simulink library "FAS"  (R2022b)
settings: Solver=VariableStepAuto  StartTime=0.0  StopTime=10.0  RelTol=1e-3
undefined symbols (not defined in the file or in its folder): FASAppl, FASComp
libraries: FasBtc x2
settings Model: Creator=sk1042978  LastModifiedBy=kl13806
settings SolverCC: AlgebraicLoopSolver=TrustRegion
settings DebuggingCC: UnconnectedInputMsg=warning  UnconnectedOutputMsg=warning  UnconnectedLineMsg=warning  SFMachineParentedDataDiag=warning
settings ModelReferenceCC: EnableRefExpFcnMdlSchedulingChecks=on
settings RTWCC: DLArmComputeVersion=19.05

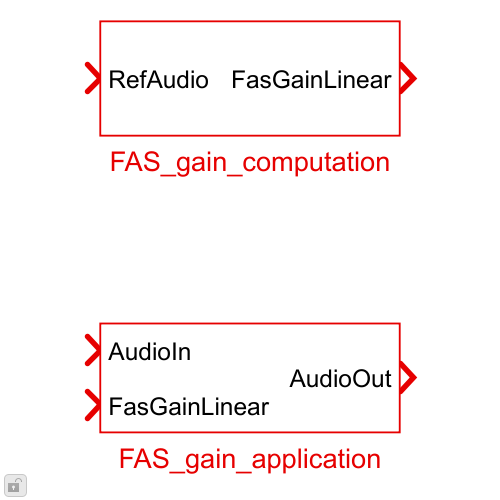
[thumbnail: Simulink's stored preview of the top-level diagram]
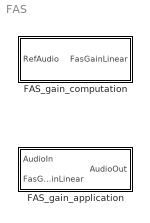
== system FAS ==
  FAS_gain_application : Subsystem  mask(Bose Fresh Air Speakers - Gain Application){MaskFasEnable=[ones(10,1)' zeros(6,1)'], MaskFASConfig=FASAppl, MaskDefaultFlag=on}
      mask prompts: MaskFasEnable "FAS enable"; MaskFASConfig "Configuration"; MaskDefaultFlag "Use default configuration"
      mask help:
      | The Fresh Air Speaker (FAS) algorithm is designed to limit the output level of selected speaker channels. The level of the remaining channels remains unaffected. This has been implemented in 2 parts - a FAS gain computation block and a FAS gain application block. Refer to the Help section for more information.
      |
      | This limiting is only necessary when windows are open, leading to a reduction in the excursion range of the FAS transducers in order to prevent damage.
      mask init:
      | blkh = gcbh;
      | 
      | % Clobber the configuration if the default values are desired
      | if (MaskDefaultFlag)
      |     MaskFASConfig = [];
      | end
      | MaskFASConfig = BTConfig.Assert('FASApplicationConfig',MaskFASConfig);
      | 
      | % Copy from MaskFASConfig to FasGainApplicationConfig
      | InnerLinkConfig = FasGainApplicationConfig;
      | InnerLinkConfig.DefaultLpfTimeConstMsec = MaskFASConfig.lpfTimeConstMsec;
      | 
      | % Copy the (previously) promoted TuneVar default to BTC
      | InnerLinkConfig.DefautFasEnable = MaskFasEnable;
      mask Help:
      | FAS Gain Application:
      | Description:
      | Applies the gain factor to the incoming audio after ramping it using a LPF. Inputs to the block are the gain factor (at framerate) and the input audio. Output from the block is the audio with the gain factors applied.
      | 
      | Mask parameters:
      | 1. FAS enable for each channel (uint32 ; [numChannels x 1]) - Either 0/1 (FAS disable/enable). Will throw an error if number of input audio channels does not match this array size.
      | 2. System parameters like frame size and sample rate are extracted from the input audio.
      | 3. Configuration: The default configuration is defined in FASApplicationConfig.m (FAS computation has a separate configuration file). Please check the file for more details on how to modify the default values.
      | 
      | Tuning support:
      | 1. LPF cut-off frequency - (Hz ; single) Ramps the gain factor
      | 2. FAS enable for each channel - (uint32) Promoted as a mask parameter
      mask Callback MaskDefaultFlag: FASMask.DefaultFlagCallback(gcbh,'MaskDefaultFlag','MaskFASConfig');
  FAS_gain_computation : Subsystem  mask(Bose Fresh Air Speakers - Gain Computation){MaskFASConfig=FASComp, MaskDefaultFlag=on}
      mask prompts: MaskFASConfig "Configuration"; MaskDefaultFlag "Use default configuration"
      mask help:
      | The Fresh Air Speaker (FAS) algorithm is designed to limit the output level of selected speaker channels. The output level of the remaining channels remains unaffected. This has been implemented in 2 parts - a FAS gain computation block and a FAS gain application block. The audio input to this block is only used to get audio stats (which will define the samplerate of this block).
      |
      | This limiting is only necessary when windows are open, leading to a reduction in the excursion range of the FAS transducers in order to prevent damage.
      mask init:
      | blkh = gcbh;
      | 
      | % Clobber the configuration if the default values are desired
      | if (MaskDefaultFlag)
      |     MaskFASConfig = [];
      | end
      | MaskFASConfig = BTConfig.Assert('FASComputationConfig',MaskFASConfig);
      | 
      | % Copy from MaskFASConfig to FasGainComputationConfig
      | InnerLinkConfig = FasGainComputationConfig;
      | InnerLinkConfig.DefaultSpeedGainSlope = MaskFASConfig.SpeedGainSlope;
      | InnerLinkConfig.DefaultSpeedGainThreshold = MaskFASConfig.SpeedGainThreshold;
      | InnerLinkConfig.DefaultGainMinValue = MaskFASConfig.GainMinValue;
      | InnerLinkConfig.DefaultSlewAttackDbPerSec = MaskFASConfig.slew_attackdBperSec;
      | InnerLinkConfig.DefaulySlewDecayDbPerSec = MaskFASConfig.slew_decaydBperSec;
      | InnerLinkConfig.DefaultSlewSlowDbPerSec = MaskFASConfig.slew_slowSlewdBperSec;
      | InnerLinkConfig.DefaultSlewThreshold = MaskFASConfig.slew_threshold;
      mask Help:
      | FAS Gain computation:
      | Description:
      | Computes the gain factor (based on speed and window status) to be applied to the channels which need pressure protection. Speed input is to be provided (either from the AudioPilot block or from a standalone RTC). The output gain factor is a value between [0,1]. System parameters like frame size and sample rate need to be provided through the mask.
      | 
      | Mask parameters:
      | 1. Configuration: The default configuration is defined in FASComputationConfig.m (FASApplication has a separate configuration file). Please check the file for more details on how to modify the default configuration.
      | 
      | Control support :
      | 1. Window Open status - (uint32) Can be 0 (window not open, FAS not needed) or 1 (window open, FAS needed).
      | 2. Speed In - (single) Current speed of the vehicle
      | 
      | Tuning support:
      | 1. Log minimum value - (single) To ensure that the computed gain in dB does not go to zero
      | 2. Slew Attack - (dB/second) Controls how fast the gain factor increases. TOP is specified in dB/samples.
      | 3. Slew Decay - (dB/second) Controls how fast the gain factor decreases. TOP is specified in dB/samples.
      | 4. Slew Threshold - (dB) If the change in slew is within this threshold, there is no update.
      | 5. Slow slew- (dB/second) Can be ignored for FAS.
      | 6. Speed Threshold (speed units) - Speed beyond which a negative gain is applied
      | 7. Speed Slope - Slope which the speed curve follows for the gain reduction.
      mask Callback MaskDefaultFlag: FASMask.DefaultFlagCallback(gcbh,'MaskDefaultFlag','MaskFASConfig');

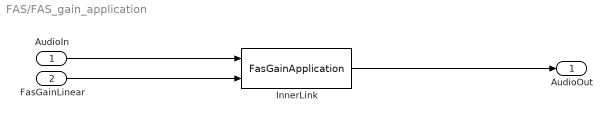
== system FAS/FAS_gain_application ==
  AudioIn : Inport
  FasGainLinear : Inport  Port=2
  InnerLink : FasBtc/FasGainApplication  Config=InnerLinkConfig  FeatureName=fas_application_
      settings: SourceProductName=Bose Blocklib
  AudioOut : Outport
  wires:
  InnerLink/1 -> AudioOut/1
  AudioIn/1 -> InnerLink/1
  FasGainLinear/1 -> InnerLink/2

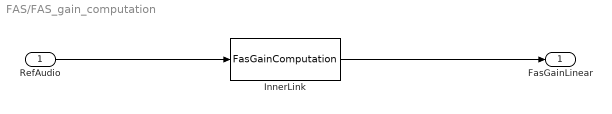
== system FAS/FAS_gain_computation ==
  RefAudio : Inport
  InnerLink : FasBtc/FasGainComputation  Config=InnerLinkConfig  FeatureName=fas_computation_
      settings: SourceProductName=Bose Blocklib
  FasGainLinear : Outport
  wires:
  InnerLink/1 -> FasGainLinear/1
  RefAudio/1 -> InnerLink/1
